simulink model "lab04part10"  (R2015a)
settings: Solver=ode45  StartTime=0.0  StopTime=50.0  RelTol=1e-3
settings Model: Creator=dg  LastModifiedBy=dg

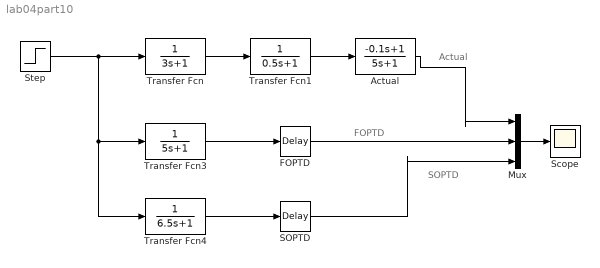
== system lab04part10 ==
  note: Actual
  note: SOPTD
  note: FOPTD
  Actual : TransferFcn  Numerator=[-0.1 1]  Denominator=[5 1]
  FOPTD : TransportDelay  DelayTime=3.6
  Mux : Mux  Inputs=3
  SOPTD : TransportDelay  DelayTime=2.1
  Scope : Scope
      settings: ShowLegends=on
  Step : Step  SampleTime=0
  Transfer Fcn : TransferFcn  Denominator=[3 1]
  Transfer Fcn1 : TransferFcn  Denominator=[0.5 1]
  Transfer Fcn3 : TransferFcn  Denominator=[5 1]
  Transfer Fcn4 : TransferFcn  Denominator=[6.5 1]
  wires:
  Step/1 -> Transfer Fcn4/1, Transfer Fcn3/1, Transfer Fcn/1
  Transfer Fcn/1 -> Transfer Fcn1/1
  Transfer Fcn1/1 -> Actual/1
  Mux/1 -> Scope/1
  Actual/1 -> Mux/1
  Transfer Fcn3/1 -> FOPTD/1
  Transfer Fcn4/1 -> SOPTD/1
  FOPTD/1 -> Mux/2
  SOPTD/1 -> Mux/3
